simulink model "Aufgabe_2 (2)"  (R2012b)
settings: Solver=ode45  StartTime=0.0  StopTime=30  RelTol=1e-3
undefined symbols (not defined in the file or in its folder): param
settings Model: Creator=stschmid  LastModifiedBy=stschmid

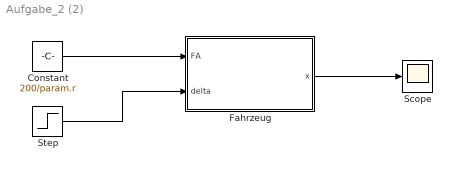
== system Aufgabe_2 (2) ==
  Constant : Constant  Value=200/param.r
  Fahrzeug : Subsystem
  Scope : Scope
  Step : Step  After=0.1  SampleTime=0
  wires:
  Fahrzeug/1(x) -> Scope/1
  Constant/1 -> Fahrzeug/1(FA)
  Step/1 -> Fahrzeug/2(delta)

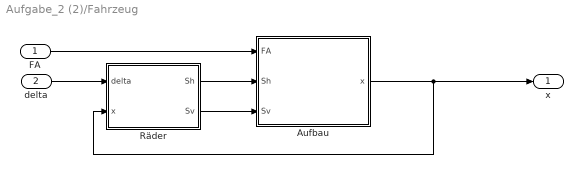
== system Aufgabe_2 (2)/Fahrzeug ==
  FA : Inport
  delta : Inport  Port=2
  Aufbau : Subsystem
  Räder : MATLAB Function  TreatAsAtomicUnit=on
  x : Outport
  wires:
  Räder/1(Sh) -> Aufbau/2(Sh)
  Aufbau/1(x) -> x/1, Räder/2(x)
  Räder/2(Sv) -> Aufbau/3(Sv)
  delta/1 -> Räder/1(delta)
  FA/1 -> Aufbau/1(FA)

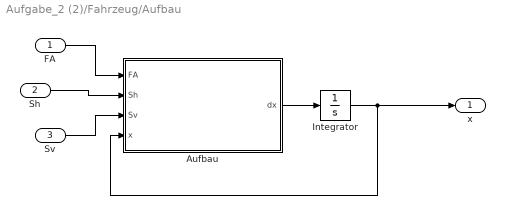
== system Aufgabe_2 (2)/Fahrzeug/Aufbau ==
  FA : Inport
  Sh : Inport  Port=2
  Sv : Inport  Port=3
  Aufbau : MATLAB Function  TreatAsAtomicUnit=on
  Integrator : Integrator  InitialCondition=zeros(6,1)
  x : Outport
  wires:
  Sh/1 -> Aufbau/2(Sh)
  Integrator/1 -> x/1, Aufbau/4(x)
  Sv/1 -> Aufbau/3(Sv)
  FA/1 -> Aufbau/1(FA)
  Aufbau/1(dx) -> Integrator/1

== matlab function Aufgabe_2 (2)/Fahrzeug/Räder ==
  data: delta input; Sh output; x input; param parameter; Sv output
function [Sh,Sv] = Raeder(delta,x,param)
%#codegen
if x(4)>0.1
alphav=x(1)-param.lv/x(4)*x(3)+delta;
alphah=x(1)+param.lh/x(4)*x(3);
else
    alphav=0;
    alphah=0;
end

Sv=param.cv*alphav;
Sh=param.ch*alphah;

== matlab function Aufgabe_2 (2)/Fahrzeug/Aufbau/Aufbau ==
  data: dx output; FA input; Sh input; Sv input; x input; param parameter
function dx = Aufbau(FA,Sh,Sv,x,param)
%#codegen
dx=zeros(6,1);
FLx=param.cL*x(4)^2;
if x(4)>0.1
dx(1)=x(3)-1/(param.m*x(4))*((FA-FLx)*x(1)+Sh+Sv);
else
dx(1)=0;
end
dx(2)=x(3);
dx(3)=1/param.Jzz*(Sv*param.lv-Sh*param.lh);
dx(4)=1/param.m*(FA-FLx);
dx(5)=x(4)*cos(x(2)-x(1));
dx(6)=x(4)*sin(x(2)-x(1));
